simulink model "chua_controlled_sim"  (R2023b)
settings: Solver=ode45  StartTime=0.0  StopTime=Tfin  RelTol=1e-3  EnableMultiTasking=on
undefined symbols (not defined in the file or in its folder): chua_circuit, k, u_bar, x0, x_bar
settings Model: Creator=s329152  LastModifiedBy=Msi
settings SolverCC: AlgebraicLoopSolver=TrustRegion
settings DataIOCC: LimitDataPoints=on  SaveFormat=Array  ReturnWorkspaceOutputs=off
settings OptimizationCC: LifeSpan=inf
settings DebuggingCC: SolverPrmCheckMsg=warning  UnconnectedInputMsg=warning  UnconnectedOutputMsg=warning  UnconnectedLineMsg=warning  SFUnexpectedBacktrackingDiag=warning  SFNoUnconditionalDefaultTransitionDiag=warning  SFExecutionAtInitializationDiag=none  ArithmeticOperatorsInVariantConditions=warning
settings HardwareCC: ProdBitPerPointer=32  ProdBitPerSizeT=32  ProdBitPerPtrDiffT=32  ProdLargestAtomicFloat=None  ProdIntDivRoundTo=Undefined  ProdEndianess=Unspecified  ProdWordSize=32  ProdHWDeviceType=32-bit Generic
settings ModelReferenceCC: PropagateSignalLabelsOutOfModel=off
settings SFSimCC: SimUseLocalCustomCode=off  CustomCodeUndefinedFunction=UseInterfaceOnly
settings RTWCC: RTWUseLocalCustomCode=off
settings CodeAppCC: StateflowObjectComments=on
settings GRTTargetCC: TargetLangStandard=C89/C90 (ANSI)
settings ConfigComp: CovMetricSettings=dw  CovSaveCumulativeToWorkspaceVar=on  CovSaveSingleToWorkspaceVar=on  CovExternalEMLEnable=off  CovSFcnEnable=off

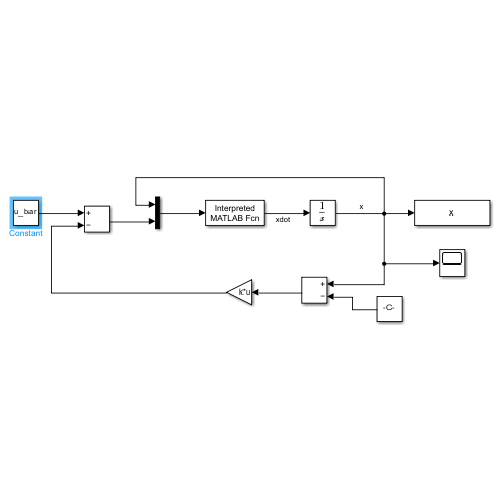
[thumbnail: Simulink's stored preview of the top-level diagram]
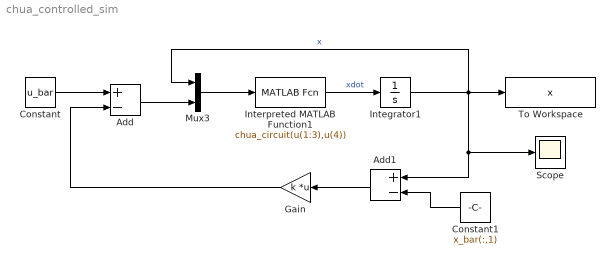
== system chua_controlled_sim ==
  Add : Sum  Inputs=+-
  Add1 : Sum  Inputs=+-
  Constant : Constant  Value=u_bar  SampleTime=0.1
  Constant1 : Constant  Value=x_bar(:,1)  SampleTime=0.1
  Gain : Gain  Gain=k  Multiplication=Matrix(K*u)
  Integrator1 : Integrator  InitialCondition=x0
  Interpreted MATLAB Function1 : MATLABFcn  MATLABFcn=chua_circuit(u(1:3),u(4))
  Mux3 : Mux  Inputs=2
  Scope : Scope
  To Workspace : ToWorkspace  VariableName=x  SampleTime=0.1
      settings: Save2DSignal=2-D array (concatenate along first dimension)
  wires:
  Interpreted MATLAB Function1/1 -> Integrator1/1  "xdot"
  Integrator1/1 -> Scope/1, Add1/1, To Workspace/1, Mux3/1  "x"
  Mux3/1 -> Interpreted MATLAB Function1/1
  Constant/1 -> Add/1
  Add/1 -> Mux3/2
  Gain/1 -> Add/2
  Add1/1 -> Gain/1
  Constant1/1 -> Add1/2
